simulink model "ThrottleArea"  (R2025b)
settings: Solver=FixedStepAuto  StartTime=0.0  StopTime=10.0  FixedStep=0.001  RelTol=1e-3
undefined symbols (not defined in the file): alpha0, alpha1
settings Model: Creator=khanh  LastModifiedBy=khanh

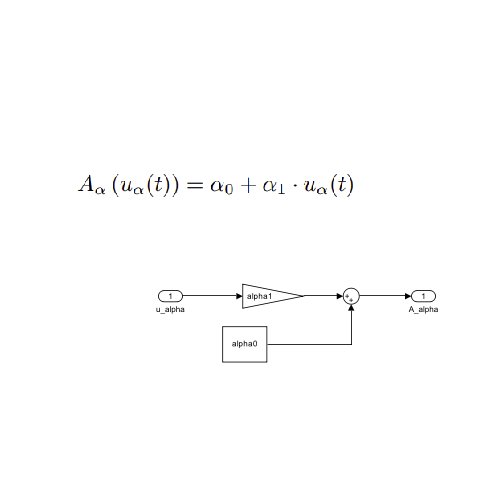
[thumbnail: Simulink's stored preview of the top-level diagram]
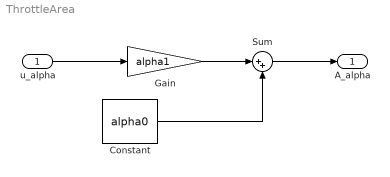
== system ThrottleArea ==
  u_alpha : Inport
  Constant : Constant  Value=alpha0
  Gain : Gain  Gain=alpha1
  Sum : Sum  Inputs=|++
  A_alpha : Outport
  wires:
  u_alpha/1 -> Gain/1
  Gain/1 -> Sum/1
  Constant/1 -> Sum/2
  Sum/1 -> A_alpha/1
